simulink model "mainECU"  (R2015b)
settings: Solver=FixedStepDiscrete  StartTime=0.0  StopTime=Inf  FixedStep=0.001  RelTol=1e-3
PostLoadFcn:
  | , if any(exist('dsrtsu_mdlpostloadfcn', 'file') == [2, 3, 6]), try dsrtsu_mdlpostloadfcn('Execute', bdroot); catch fprintf('Error in PostLoadFcn (dsrtsu_mdlpostloadfcn) for model "%s":\n %s\n', bdroot, lasterr); end, end,
undefined symbols (not defined in the file or in its folder): STARTUP
libraries: dspswit3 x5, rtican x5, simulink x2
(part 2 of 2)

== system mainECU/RTI Data/RTI Data Store/RTI Data Store ==
  RTI Data Store : Subsystem  mask(RTI_DATA_STORE){}
      mask help:
      | RTI Data Store Block. This block is used by RTI to store internal model dependent data. Deleting this block will result in data loss.
      |
      | NEVER DELETE, COPY, OR MODIFY THIS BLOCK!
      mask Help:
      | RTI Data Store Block. This block is used by RTI to store internal model dependent data. Deleting this block will result in data loss.
      | 
      | NEVER DELETE, COPY, OR MODIFY THIS BLOCK!
      mask Display: text(0.5, 0.5, ' ', 'HorizontalAlignment', 'center');

== system mainECU/RTI Data/RTI Data Store/RTI Data Store/RTI Data Store ==
  RTI Data Store : Subsystem  mask(RTI_DATA_STORE){}
      mask help:
      | RTI Data Store Block. This block is used by RTI to store internal model dependent data. Deleting this block will result in data loss.
      |
      | NEVER DELETE, COPY, OR MODIFY THIS BLOCK!
      mask Help:
      | RTI Data Store Block. This block is used by RTI to store internal model dependent data. Deleting this block will result in data loss.
      | 
      | NEVER DELETE, COPY, OR MODIFY THIS BLOCK!
      mask Display: text(0.5, 0.5, ' ', 'HorizontalAlignment', 'center');

== system mainECU/RTI Data/RTI Data Store/RTI Data Store/RTI Data Store/RTI Data Store ==

== stateflow chart mainECU/Chart ==
  state Startup
    entry:
    power_mode = STARTUP
    during:
    exit:
  note: Startup
      | Sequence
  state Idle
    entry:
    power_mode = IDLE
    during:
    exit:
  state ReadyToDrive
    entry:
    power_mode = RTD
    during:
    exit:
  note: Non critical fault
      | Recovered
  note: Fault
      | Detected
  state Stopped
    entry:
    power_mode = STOPPED
    during:
    exit:
  state Fault
    entry:
    power_mode = FAULTED
    during:
    exit:
  note: Critical Fault
      | Detected
  (default) -> Startup
  Startup -> Idle : after(2,sec)
  Idle -> ReadyToDrive [order 1] : [brake > 90 && klemme15 == 1 && diagnosticStatus ~= 1]
  ReadyToDrive -> Fault
  Fault -> ReadyToDrive [order 1]
  Idle -> Stopped [order 2] : [diagnosticStatus == 1]
  Stopped -> Idle : [diagnosticStatus ~= 1]
  Fault -> Stopped [order 2]
  data: power_mode output double =0; brake input [0..100]; klemme15 input; diagnosticStatus input; IDLE constant double =0; STOPPED constant double =1; RTD constant double =2; FAULTED constant double =3; STARTUP constant double =4
